simulink model "vdpStateEstimationModel"  (R2018a)
settings: Solver=VariableStepAuto  StartTime=0.0  StopTime=5  RelTol=1e-3
libraries: simulink x1, sharedTrackingLibrary x1
settings Model: Creator=The MathWorks, Inc.  LastModifiedBy=The MathWorks, Inc.
settings CodeAppCC: StateflowObjectComments=on

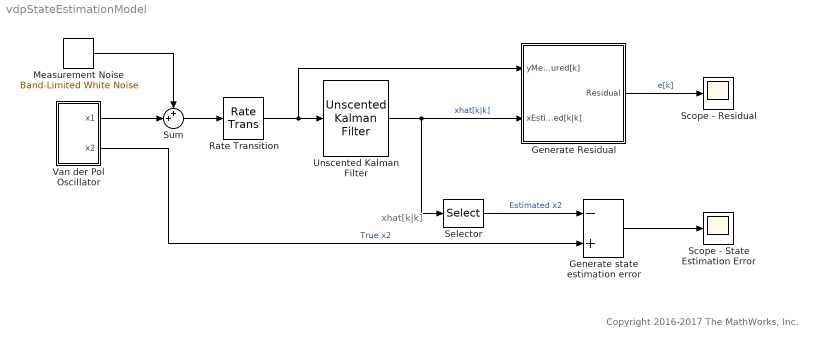
== system vdpStateEstimationModel ==
  note: xhat[k|k]
  note: Copyright 2016-2017 The MathWorks, Inc.
  Generate Residual : Subsystem
  Generate state estimation error : Sum  Inputs=-+
  Measurement Noise : simulink/Sources/Band-Limited White Noise  Cov=4e-4  Ts=0.05  seed=[23342]
  Rate Transition : RateTransition  OutPortSampleTime=0.05
  Scope - Residual : Scope
  Scope - State Estimation Error : Scope
  Selector : Selector  InputPortWidth=2  IndexOptions=Index vector (dialog)  Indices=2  OutputSizes=1
  Sum : Sum  Inputs=++|
  Unscented Kalman Filter : sharedTrackingLibrary/Unscented Kalman Filter  StateTransitionFcn=vdpStateFcn  HasAdditiveProcessNoise=Additive  ProcessNoise=0.1  HasTimeVaryingProcessNoise=off  HasStateTransitionFcnExtraArgument=0  InitialState=[2; 0]  InitialStateCovariance=0.1  Alpha=1e-3  Beta=2  Kappa=0  MeasurementFcn1=vdpMeasurementFcn  HasMeasurementEnablePort1=off  HasAdditiveMeasurementNoise1=Additive  MeasurementNoise1=0.05  HasTimeVaryingMeasurementNoise1=off  HasMeasurementFcnExtraArgument1=0  MeasurementFcn2=myMeasurementFcn  HasMeasurementEnablePort2=off  HasAdditiveMeasurementNoise2=Additive  MeasurementNoise2=1  HasTimeVaryingMeasurementNoise2=off  HasMeasurementFcnExtraArgument2=0  MeasurementFcn3=myMeasurementFcn  HasMeasurementEnablePort3=off  HasAdditiveMeasurementNoise3=Additive  MeasurementNoise3=1  HasTimeVaryingMeasurementNoise3=off  HasMeasurementFcnExtraArgument3=0  MeasurementFcn4=myMeasurementFcn  HasMeasurementEnablePort4=off  HasAdditiveMeasurementNoise4=Additive  MeasurementNoise4=1  HasTimeVaryingMeasurementNoise4=off  HasMeasurementFcnExtraArgument4=0  MeasurementFcn5=myMeasurementFcn  HasMeasurementEnablePort5=off  HasAdditiveMeasurementNoise5=Additive  MeasurementNoise5=1  HasTimeVaryingMeasurementNoise5=off  HasMeasurementFcnExtraArgument5=0  EnableMultirate=off  StateTransitionFcnSampleTime=1  MeasurementFcn1SampleTime=1  MeasurementFcn2SampleTime=1  MeasurementFcn3SampleTime=1  MeasurementFcn4SampleTime=1  MeasurementFcn5SampleTime=1  UseCurrentEstimator=on  OutputStateCovariance=off  DataType=double  SampleTime=0.05  NumberOfMeasurements=1
      settings: SourceProductName=Control System Toolbox  SourceProductBaseCode=CT
  Van der Pol Oscillator : Subsystem
  wires:
  Unscented Kalman Filter/1 -> Generate Residual/2(xEstimated[k|k]), Selector/1  "xhat[k|k]"
  Sum/1 -> Rate Transition/1
  Van der Pol Oscillator/1(x1) -> Sum/2
  Measurement Noise/1 -> Sum/1
  Selector/1 -> Generate state estimation error/1  "Estimated x2"
  Van der Pol Oscillator/2(x2) -> Generate state estimation error/2  "True x2"
  Generate Residual/1(Residual) -> Scope - Residual/1  "e[k]"
  Rate Transition/1 -> Unscented Kalman Filter/1, Generate Residual/1(yMeasured[k])
  Generate state estimation error/1 -> Scope - State Estimation Error/1

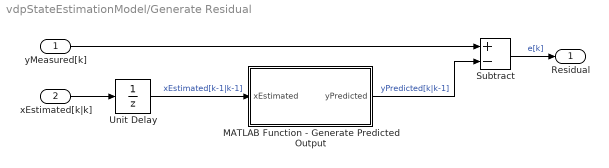
== system vdpStateEstimationModel/Generate Residual ==
  yMeasured[k] : Inport
  xEstimated[k|k] : Inport  Port=2
  MATLAB Function - Generate Predicted Output : MATLAB Function  TreatAsAtomicUnit=on
  Subtract : Sum  Inputs=+-
  Unit Delay : UnitDelay  InitialCondition=[2;0]  SampleTime=-1
  Residual : Outport
  wires:
  xEstimated[k|k]/1 -> Unit Delay/1
  Unit Delay/1 -> MATLAB Function - Generate Predicted Output/1(xEstimated)  "xEstimated[k-1|k-1]"
  MATLAB Function - Generate Predicted Output/1(yPredicted) -> Subtract/2  "yPredicted[k|k-1]"
  Subtract/1 -> Residual/1  "e[k]"
  yMeasured[k]/1 -> Subtract/1

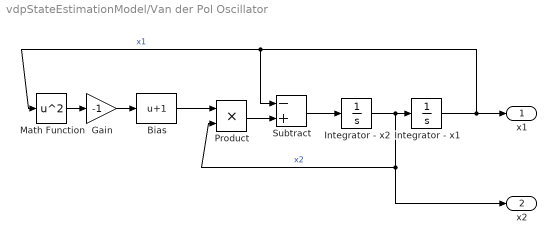
== system vdpStateEstimationModel/Van der Pol Oscillator ==
  Bias : Bias  Bias=1
  Gain : Gain  Gain=-1
  Integrator - x1 : Integrator  InitialCondition=2
  Integrator - x2 : Integrator
  Math Function : Math  Operator=square  SaturateOnIntegerOverflow=on
  Product : Product
  Subtract : Sum  Inputs=-+
  x1 : Outport
  x2 : Outport  Port=2
  wires:
  Integrator - x1/1 -> x1/1, Subtract/1, Math Function/1  "x1"
  Product/1 -> Subtract/2
  Integrator - x2/1 -> x2/1, Product/2, Integrator - x1/1  "x2"
  Subtract/1 -> Integrator - x2/1
  Gain/1 -> Bias/1
  Math Function/1 -> Gain/1
  Bias/1 -> Product/1

== matlab function vdpStateEstimationModel/Generate Residual/MATLAB Function - Generate Predicted Output ==
  data: xEstimated input; yPredicted output
function yPredicted = generatePredictedOutput(xEstimated)

%   Copyright 2017 The MathWorks, Inc.

%#codegen

% Given state estimates at previous time (k-1) utilizing measurements up to
% (k-1), predict states at current step.
xPredicted = vdpStateFcn(xEstimated); % xhat[k|k-1]
% Generate output estimate, again without utilizing the measurement at
% current time.
yPredicted = vdpMeasurementFcn(xPredicted); % y[k|k-1]
end
